simulink library "bcbLibrary"  (R2019a)
settings: Solver=VariableStepAuto  StartTime=0.0  StopTime=10.0  RelTol=1e-3
settings Model: Creator=ggparker  LastModifiedBy=vmali

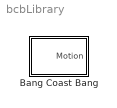
== system bcbLibrary ==
  Bang Coast Bang : Subsystem  mask{spdIC=0, posIC=0, amp=0, tPW=2, tCoast=0, tStart=1}
      mask prompts: spdIC "Speed"; posIC "Position"; amp "Accel Amp (m/s^2)"; tPW "Pulse Width (sec)"; tCoast "Coast Time (sec)"; tStart "Start Time (sec)"
      settings: AttributesFormatString=t = %<tStart>, A = %<amp>
      mask DialogControl Container12 Prompt: Initial Conditions
      mask DialogControl Container15 Prompt: Motion

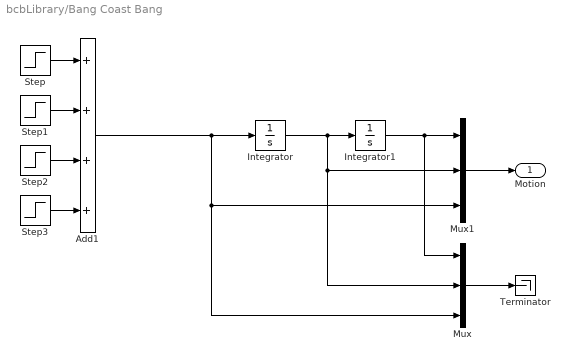
== system bcbLibrary/Bang Coast Bang ==
  Add1 : Sum  Inputs=++++
  Integrator : Integrator  InitialCondition=spdIC
  Integrator1 : Integrator  InitialCondition=posIC
  Mux : Mux  Inputs=3
  Mux1 : Mux  Inputs=3
  Step : Step  Time=tStart  After=amp  SampleTime=0
  Step1 : Step  Time=tStart+tPW  After=-amp  SampleTime=0
  Step2 : Step  Time=tStart+tPW+tCoast  After=-amp  SampleTime=0
  Step3 : Step  Time=tStart+2*tPW+tCoast  After=amp  SampleTime=0
  Terminator : Terminator
  Motion : Outport
  wires:
  Step/1 -> Add1/1
  Step1/1 -> Add1/2
  Step2/1 -> Add1/3
  Step3/1 -> Add1/4
  Add1/1 -> Integrator/1, Mux1/3, Mux/3
  Integrator/1 -> Mux1/2, Mux/2, Integrator1/1
  Integrator1/1 -> Mux1/1, Mux/1
  Mux/1 -> Terminator/1
  Mux1/1 -> Motion/1
